simulink model "ModelPID"  (R2020a)
settings: Solver=VariableStepAuto  StartTime=0.0  StopTime=10.0  RelTol=1e-3
settings Model: Creator=63586572  LastModifiedBy=63586572

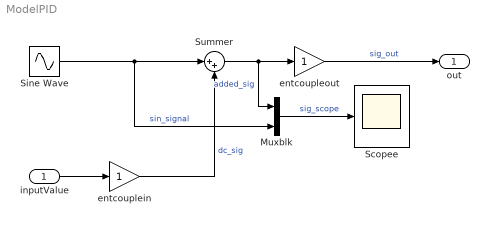
== system ModelPID ==
  inputValue : Inport
  Muxblk : Mux  Inputs=2
  Scopee : Scope
  Sine Wave : Sin  Amplitude=10  SampleTime=0
  Summer : Sum  Inputs=|++
  entcouplein : Gain
  entcoupleout : Gain
  out : Outport
  wires:
  Sine Wave/1 -> Muxblk/2, Summer/1  "sin_signal"
  inputValue/1 -> entcouplein/1
  Summer/1 -> Muxblk/1, entcoupleout/1  "added_sig"
  Muxblk/1 -> Scopee/1  "sig_scope"
  entcouplein/1 -> Summer/2  "dc_sig"
  entcoupleout/1 -> out/1  "sig_out"
